simulink model "model"  (R2023a)
settings: Solver=ode15s  StartTime=0.0  StopTime=10.0  RelTol=1e-3
values from neighbouring files (symbols this model uses):
  Jdv = 7e-6    (= 7e-06)    [script.m]
  K1 = Cm * Lov    (= 0.0169)    [script.m]
  T1 = ( Lov + Lya ) / Rya    (= 0.0035)    [script.m]
  Uupr = 10    [script.m]
undefined symbols (not defined in the file or in its folder): b
settings Model: Creator=stanc  LastModifiedBy=stanc

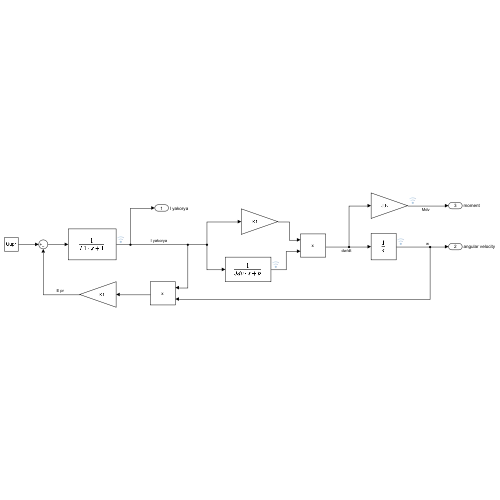
[thumbnail: Simulink's stored preview of the top-level diagram]
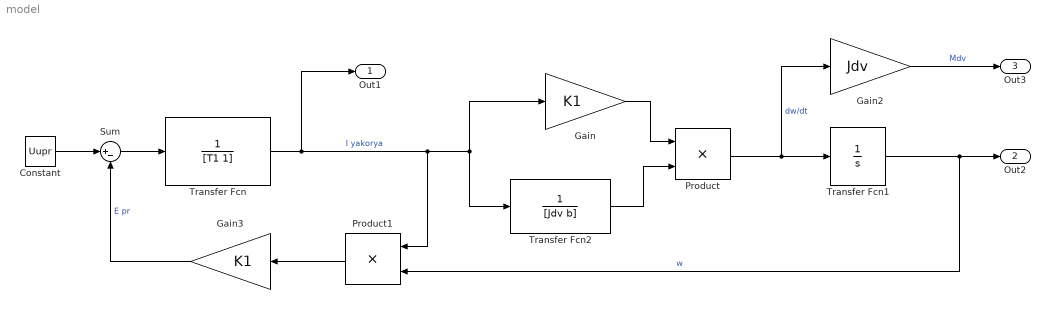
== system model ==
  Constant : Constant  Value=Uupr
  Gain : Gain  Gain=K1
  Gain2 : Gain  Gain=Jdv
  Gain3 : Gain  Gain=K1
  Product : Product
  Product1 : Product
  Sum : Sum  Inputs=|+-
  Transfer Fcn : TransferFcn  Denominator=[T1 1]
  Transfer Fcn1 : TransferFcn  Denominator=[1 0]
  Transfer Fcn2 : TransferFcn  Denominator=[Jdv b]
  Out1 : Outport  SignalName=I yakorya
  Out2 : Outport  Port=2  SignalName=angular velocity
  Out3 : Outport  Port=3  SignalName=moment
  wires:
  Transfer Fcn/1 -> Out1/1, Product1/1, Transfer Fcn2/1, Gain/1  "I yakorya"
  Sum/1 -> Transfer Fcn/1
  Constant/1 -> Sum/1
  Transfer Fcn2/1 -> Product/2
  Gain/1 -> Product/1
  Product/1 -> Transfer Fcn1/1, Gain2/1  "dw/dt"
  Transfer Fcn1/1 -> Out2/1, Product1/2  "w"
  Gain2/1 -> Out3/1  "Mdv"
  Product1/1 -> Gain3/1
  Gain3/1 -> Sum/2  "E pr"
